simulink model "ReadAnalogInput"  (Simulink 7.7)
settings: Solver=FixedStepDiscrete  StartTime=0.0  StopTime=60*60  FixedStep=0.001  RelTol=1e-3
InitFcn:
  | n=2;
  | Wn=20/500;
  | [Aa1,Bb1,Cc1,Dd1]=butter(n,Wn,'low')
undefined symbols (not defined in the file or in its folder): Aa1, Bb1, Cc1, Dd1
libraries: Diamond16AT_UNAL x1
settings Model: Creator=LAB_Mecatronica_16  LastModifiedBy=Edgar  SimulationMode=external  BufferReuse=off
settings DataIOCC: LimitDataPoints=off
settings OptimizationCC: BlockReduction=off  OptimizeBlockIOStorage=off  BufferReuse=off  ExpressionFolding=off  LocalBlockOutputs=off
settings HardwareCC: ProdIntDivRoundTo=Zero  ProdEndianess=LittleEndian  ProdHWDeviceType=Generic->32-bit x86 compatible
settings RTWCC: SystemTargetFile=xpctarget.tlc  TemplateMakefile=xpc_default_tmf  Description=xPC Target  ProcessScript=xpctarget_make_rtw_hook  RTWCompilerOptimization=On
settings xpcTargetCC: TargetFcnLib=ansi_tfl_table_tmw.mat  TargetFunctionLibrary=XPC_BLAS  FunctionExecutionProfile=off  CodeExecutionProfiling=off  ERTCodeCoverageTool=None  ParMdlRefBuildCompliant=on  CombineSignalStateStructs=off  PortableWordSizes=off  RL32LogBufSizeModifier=15000000  xPCTaskExecutionProfile=off  xPCRL32EventNumber=5000  xPCLoadParamSetFile=off  xPCConcurrentTasks=off  xPCEnableSFAnimation=off

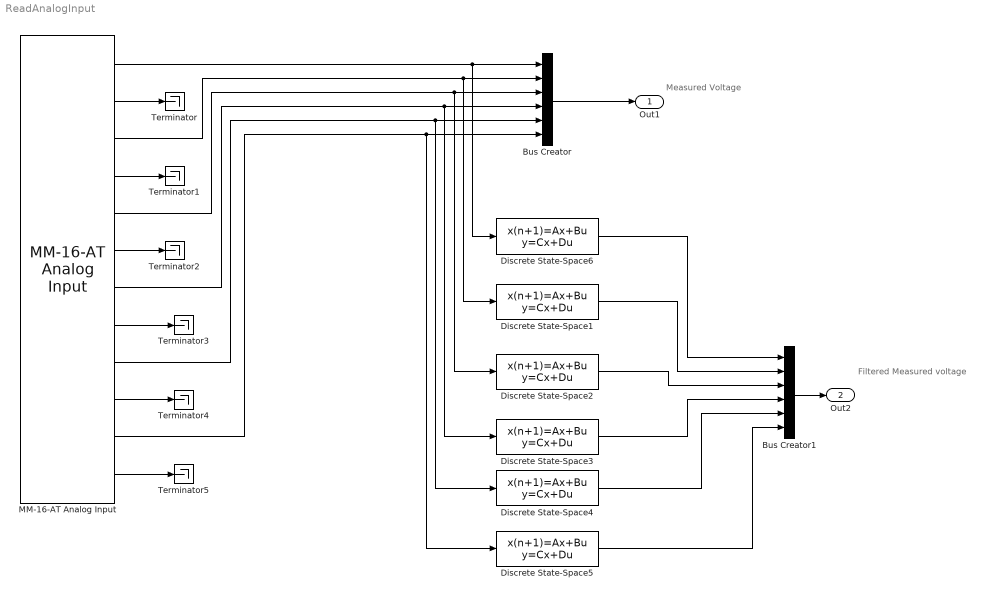
== system ReadAnalogInput ==
  note: Measured Voltage
  note: Filtered Measured voltage
  Bus Creator : BusCreator  Inputs=6
  Bus Creator1 : BusCreator  Inputs=6
  Discrete State-Space{1..6} (6 alike) : DiscreteStateSpace  A=Aa1  B=Bb1  C=Cc1  D=Dd1  X0=[0 0]  SampleTime=-1
  MM-16-AT Analog Input : Diamond16AT_UNAL/Diamond MM-16-AT/MM-16-AT Analog Input  configuration=16 Single-ended  firstChan=1  numChans=12  range=0 to 5V  sampleTime=0.001  base=300
  Terminator{,1..5} (6 alike) : Terminator
  Out1 : Outport
  Out2 : Outport  Port=2
  wires:
  Discrete State-Space6/1 -> Bus Creator1/1
  Discrete State-Space1/1 -> Bus Creator1/2
  Discrete State-Space2/1 -> Bus Creator1/3
  Discrete State-Space3/1 -> Bus Creator1/4
  Discrete State-Space4/1 -> Bus Creator1/5
  Discrete State-Space5/1 -> Bus Creator1/6
  Bus Creator1/1 -> Out2/1
  Bus Creator/1 -> Out1/1
  MM-16-AT Analog Input/1 -> Bus Creator/1, Discrete State-Space6/1
  MM-16-AT Analog Input/3 -> Bus Creator/2, Discrete State-Space1/1
  MM-16-AT Analog Input/5 -> Bus Creator/3, Discrete State-Space2/1
  MM-16-AT Analog Input/7 -> Bus Creator/4, Discrete State-Space3/1
  MM-16-AT Analog Input/9 -> Bus Creator/5, Discrete State-Space4/1
  MM-16-AT Analog Input/11 -> Bus Creator/6, Discrete State-Space5/1
  MM-16-AT Analog Input/2 -> Terminator/1
  MM-16-AT Analog Input/4 -> Terminator1/1
  MM-16-AT Analog Input/6 -> Terminator2/1
  MM-16-AT Analog Input/8 -> Terminator3/1
  MM-16-AT Analog Input/10 -> Terminator4/1
  MM-16-AT Analog Input/12 -> Terminator5/1
